simulink model "HW2_1_disc"  (R2021a)
settings: Solver=VariableStepAuto  StartTime=0.0  StopTime=10  RelTol=1e-3
settings Model: Creator=jhart  LastModifiedBy=jhart

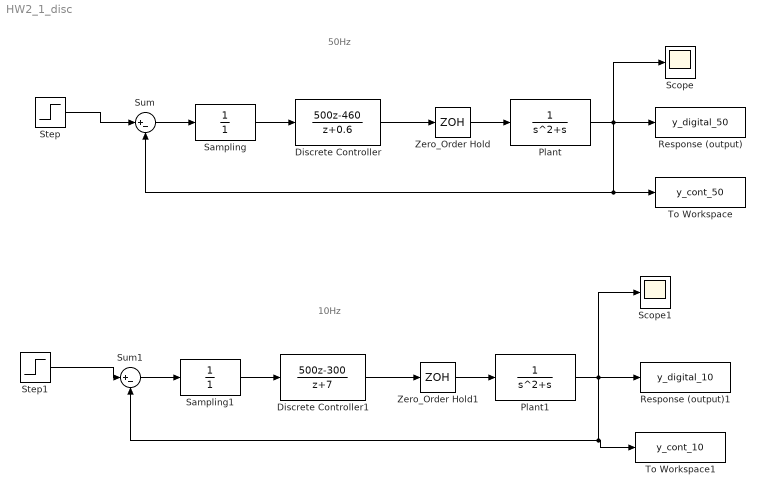
== system HW2_1_disc ==
  note: 50Hz
  note: 10Hz
  Discrete Controller : DiscreteTransferFcn  Numerator=[500 -460]  Denominator=[1 0.6]  SampleTime=0.02
  Discrete Controller1 : DiscreteTransferFcn  Numerator=[500 -300]  Denominator=[1 7]  SampleTime=0.1
  Plant : TransferFcn  Denominator=[1 1 0]
  Plant1 : TransferFcn  Denominator=[1 1 0]
  Response (output) : ToWorkspace  VariableName=y_digital_50  SaveFormat=Timeseries  SampleTime=0.02
  Response (output)1 : ToWorkspace  VariableName=y_digital_10  SaveFormat=Timeseries  SampleTime=0.1
  Sampling : DiscreteTransferFcn  Denominator=[1]  SampleTime=0.02
  Sampling1 : DiscreteTransferFcn  Denominator=[1]  SampleTime=0.1
  Scope : Scope
  Scope1 : Scope
  Step : Step  Time=0  SampleTime=0
  Step1 : Step  Time=0  SampleTime=0
  Sum : Sum  Inputs=|+-
  Sum1 : Sum  Inputs=|+-
  To Workspace : ToWorkspace  VariableName=y_cont_50  SaveFormat=Timeseries  SampleTime=-1
  To Workspace1 : ToWorkspace  VariableName=y_cont_10  SaveFormat=Timeseries  SampleTime=-1
  Zero_Order Hold : ZeroOrderHold  SampleTime=0.02
  Zero_Order Hold1 : ZeroOrderHold  SampleTime=0.1
  wires:
  Discrete Controller/1 -> Zero_Order Hold/1
  Sum/1 -> Sampling/1
  Zero_Order Hold/1 -> Plant/1
  Sampling/1 -> Discrete Controller/1
  Step/1 -> Sum/1
  Sum1/1 -> Sampling1/1
  Sampling1/1 -> Discrete Controller1/1
  Plant1/1 -> Scope1/1, Sum1/2, To Workspace1/1, Response (output)1/1
  Discrete Controller1/1 -> Zero_Order Hold1/1
  Zero_Order Hold1/1 -> Plant1/1
  Plant/1 -> Scope/1, Sum/2, To Workspace/1, Response (output)/1
  Step1/1 -> Sum1/1
